simulink model "project"  (R2018b)
settings: Solver=VariableStepAuto  StartTime=0.0  StopTime=10.0  RelTol=1e-3
libraries: commutil2 x4
(part 1 of 2)
settings Model: Creator=Reza  LastModifiedBy=Rahmat

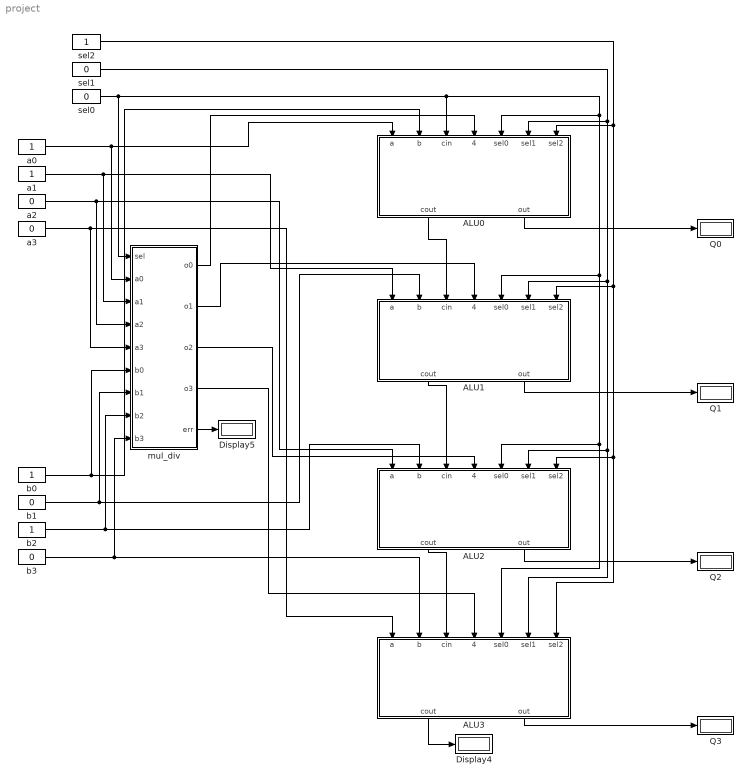
== system project ==
  ALU0 : Subsystem
  ALU1 : Subsystem
  ALU2 : Subsystem
  ALU3 : Subsystem
  Display4 : Display
  Display5 : Display
  Q{0..3} (4 alike) : Display
  a0 : Constant
  a1 : Constant
  a2 : Constant  Value=0
  a3 : Constant  Value=0
  b0 : Constant
  b1 : Constant  Value=0
  b2 : Constant
  b3 : Constant  Value=0
  mul_div : Subsystem
  sel0 : Constant  Value=0
  sel1 : Constant  Value=0
  sel2 : Constant
  wires:
  mul_div/1(o0) -> ALU0/4(mul_div)
  mul_div/2(o1) -> ALU1/4(mul_div)
  mul_div/3(o2) -> ALU2/4(mul_div)
  mul_div/4(o3) -> ALU3/4(mul_div)
  ALU0/1(cout) -> ALU1/3(cin)
  ALU1/1(cout) -> ALU2/3(cin)
  ALU2/1(cout) -> ALU3/3(cin)
  ALU0/2(out) -> Q0/1
  ALU1/2(out) -> Q1/1
  ALU2/2(out) -> Q2/1
  ALU3/2(out) -> Q3/1
  ALU3/1(cout) -> Display4/1
  mul_div/5(err) -> Display5/1
  sel0/1 -> mul_div/1(sel), ALU0/3(cin), ALU0/5(sel0), ALU1/5(sel0), ALU3/5(sel0), ALU2/5(sel0)
  sel1/1 -> ALU0/6(sel1), ALU1/6(sel1), ALU2/6(sel1), ALU3/6(sel1)
  sel2/1 -> ALU0/7(sel2), ALU1/7(sel2), ALU2/7(sel2), ALU3/7(sel2)
  a0/1 -> ALU0/1(a), mul_div/2(a0)
  a1/1 -> mul_div/3(a1), ALU1/1(a)
  a2/1 -> mul_div/4(a2), ALU2/1(a)
  a3/1 -> mul_div/5(a3), ALU3/1(a)
  b0/1 -> ALU0/2(b), mul_div/6(b0)
  b1/1 -> ALU1/2(b), mul_div/7(b1)
  b2/1 -> ALU2/2(b), mul_div/8(b2)
  b3/1 -> ALU3/2(b), mul_div/9(b3)

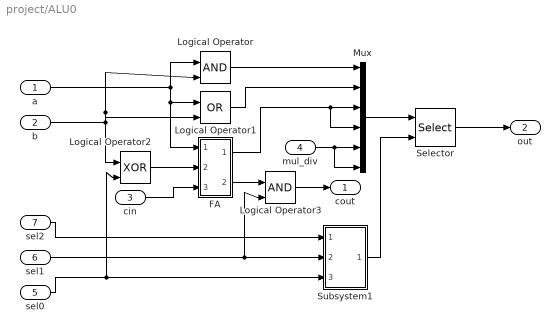
== system project/ALU0 ==
  a : Inport
  b : Inport  Port=2
  cin : Inport  Port=3
  mul_div : Inport  Port=4
  sel0 : Inport  Port=5
  sel1 : Inport  Port=6
  sel2 : Inport  Port=7
  FA : Subsystem
  Logical Operator : Logic  IconShape=distinctive  AllPortsSameDT=off  OutDataTypeStr=boolean
  Logical Operator1 : Logic  Operator=OR  IconShape=distinctive  AllPortsSameDT=off  OutDataTypeStr=boolean
  Logical Operator2 : Logic  Operator=XOR  IconShape=distinctive  AllPortsSameDT=off  OutDataTypeStr=boolean
  Logical Operator3 : Logic  IconShape=distinctive  AllPortsSameDT=off  OutDataTypeStr=boolean
  Mux : Mux  Inputs=6
  Selector : Selector  InputPortWidth=6  IndexOptions=Starting index (port)  Indices=[1 3]  OutputSizes=1
  Subsystem1 : Subsystem
  cout : Outport
  out : Outport  Port=2
  wires:
  b/1 -> Logical Operator/2, Logical Operator1/2, Logical Operator2/1
  Mux/1 -> Selector/1
  sel1/1 -> Logical Operator3/2, Subsystem1/2(sel1)
  FA/1(Out2) -> Mux/3, Mux/4
  sel2/1 -> Subsystem1/1(sel2)
  Subsystem1/1(Out1) -> Selector/2
  a/1 -> FA/1(In2), Logical Operator1/1, Logical Operator/1
  cin/1 -> FA/3(In4)
  Logical Operator2/1 -> FA/2(In3)
  Selector/1 -> out/1
  sel0/1 -> Logical Operator2/2, Subsystem1/3(sel0)
  Logical Operator1/1 -> Mux/2
  Logical Operator/1 -> Mux/1
  mul_div/1 -> Mux/5, Mux/6
  FA/2(Out1) -> Logical Operator3/1
  Logical Operator3/1 -> cout/1

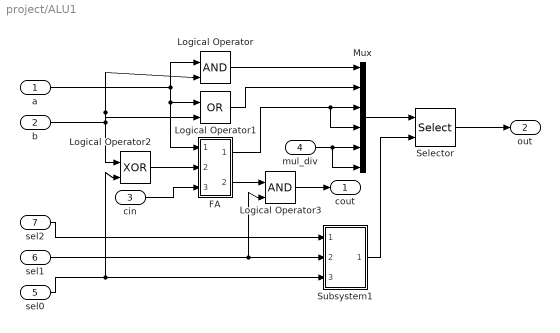
== system project/ALU1 ==
  a : Inport
  b : Inport  Port=2
  cin : Inport  Port=3
  mul_div : Inport  Port=4
  sel0 : Inport  Port=5
  sel1 : Inport  Port=6
  sel2 : Inport  Port=7
  FA : Subsystem
  Logical Operator : Logic  IconShape=distinctive  AllPortsSameDT=off  OutDataTypeStr=boolean
  Logical Operator1 : Logic  Operator=OR  IconShape=distinctive  AllPortsSameDT=off  OutDataTypeStr=boolean
  Logical Operator2 : Logic  Operator=XOR  IconShape=distinctive  AllPortsSameDT=off  OutDataTypeStr=boolean
  Logical Operator3 : Logic  IconShape=distinctive  AllPortsSameDT=off  OutDataTypeStr=boolean
  Mux : Mux  Inputs=6
  Selector : Selector  InputPortWidth=6  IndexOptions=Starting index (port)  Indices=[1 3]  OutputSizes=1
  Subsystem1 : Subsystem
  cout : Outport
  out : Outport  Port=2
  wires:
  b/1 -> Logical Operator/2, Logical Operator1/2, Logical Operator2/1
  Mux/1 -> Selector/1
  sel1/1 -> Logical Operator3/2, Subsystem1/2(sel1)
  FA/1(Out2) -> Mux/4, Mux/3
  sel2/1 -> Subsystem1/1(sel2)
  Subsystem1/1(Out1) -> Selector/2
  a/1 -> FA/1(In2), Logical Operator1/1, Logical Operator/1
  cin/1 -> FA/3(In4)
  sel0/1 -> Logical Operator2/2, Subsystem1/3(sel0)
  Logical Operator2/1 -> FA/2(In3)
  Selector/1 -> out/1
  Logical Operator/1 -> Mux/1
  Logical Operator1/1 -> Mux/2
  mul_div/1 -> Mux/6, Mux/5
  FA/2(Out1) -> Logical Operator3/1
  Logical Operator3/1 -> cout/1

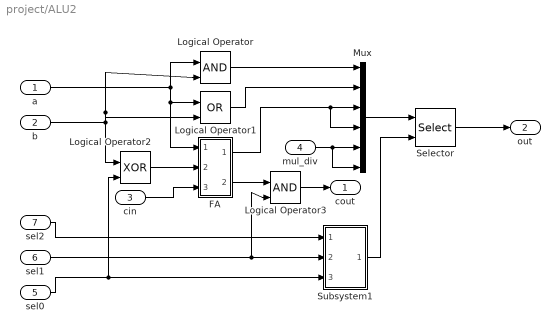
== system project/ALU2 ==
  a : Inport
  b : Inport  Port=2
  cin : Inport  Port=3
  mul_div : Inport  Port=4
  sel0 : Inport  Port=5
  sel1 : Inport  Port=6
  sel2 : Inport  Port=7
  FA : Subsystem
  Logical Operator : Logic  IconShape=distinctive  AllPortsSameDT=off  OutDataTypeStr=boolean
  Logical Operator1 : Logic  Operator=OR  IconShape=distinctive  AllPortsSameDT=off  OutDataTypeStr=boolean
  Logical Operator2 : Logic  Operator=XOR  IconShape=distinctive  AllPortsSameDT=off  OutDataTypeStr=boolean
  Logical Operator3 : Logic  IconShape=distinctive  AllPortsSameDT=off  OutDataTypeStr=boolean
  Mux : Mux  Inputs=6
  Selector : Selector  InputPortWidth=6  IndexOptions=Starting index (port)  Indices=[1 3]  OutputSizes=1
  Subsystem1 : Subsystem
  cout : Outport
  out : Outport  Port=2
  wires:
  b/1 -> Logical Operator/2, Logical Operator1/2, Logical Operator2/1
  Mux/1 -> Selector/1
  sel1/1 -> Logical Operator3/2, Subsystem1/2(sel1)
  FA/1(Out2) -> Mux/4, Mux/3
  sel2/1 -> Subsystem1/1(sel2)
  Subsystem1/1(Out1) -> Selector/2
  a/1 -> FA/1(In2), Logical Operator1/1, Logical Operator/1
  cin/1 -> FA/3(In4)
  sel0/1 -> Logical Operator2/2, Subsystem1/3(sel0)
  Logical Operator2/1 -> FA/2(In3)
  Selector/1 -> out/1
  Logical Operator1/1 -> Mux/2
  Logical Operator/1 -> Mux/1
  mul_div/1 -> Mux/5, Mux/6
  Logical Operator3/1 -> cout/1
  FA/2(Out1) -> Logical Operator3/1

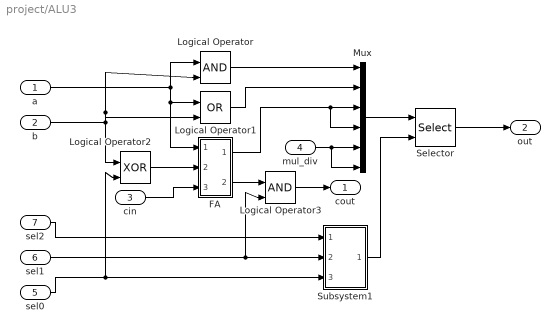
== system project/ALU3 ==
  a : Inport
  b : Inport  Port=2
  cin : Inport  Port=3
  mul_div : Inport  Port=4
  sel0 : Inport  Port=5
  sel1 : Inport  Port=6
  sel2 : Inport  Port=7
  FA : Subsystem
  Logical Operator : Logic  IconShape=distinctive  AllPortsSameDT=off  OutDataTypeStr=boolean
  Logical Operator1 : Logic  Operator=OR  IconShape=distinctive  AllPortsSameDT=off  OutDataTypeStr=boolean
  Logical Operator2 : Logic  Operator=XOR  IconShape=distinctive  AllPortsSameDT=off  OutDataTypeStr=boolean
  Logical Operator3 : Logic  IconShape=distinctive  AllPortsSameDT=off  OutDataTypeStr=boolean
  Mux : Mux  Inputs=6
  Selector : Selector  InputPortWidth=6  IndexOptions=Starting index (port)  Indices=[1 3]  OutputSizes=1
  Subsystem1 : Subsystem
  cout : Outport
  out : Outport  Port=2
  wires:
  b/1 -> Logical Operator/2, Logical Operator1/2, Logical Operator2/1
  Mux/1 -> Selector/1
  sel1/1 -> Logical Operator3/2, Subsystem1/2(sel1)
  FA/1(Out2) -> Mux/4, Mux/3
  sel2/1 -> Subsystem1/1(sel2)
  Subsystem1/1(Out1) -> Selector/2
  a/1 -> FA/1(In2), Logical Operator1/1, Logical Operator/1
  cin/1 -> FA/3(In4)
  sel0/1 -> Logical Operator2/2, Subsystem1/3(sel0)
  Logical Operator2/1 -> FA/2(In3)
  Selector/1 -> out/1
  Logical Operator1/1 -> Mux/2
  Logical Operator/1 -> Mux/1
  mul_div/1 -> Mux/6, Mux/5
  Logical Operator3/1 -> cout/1
  FA/2(Out1) -> Logical Operator3/1

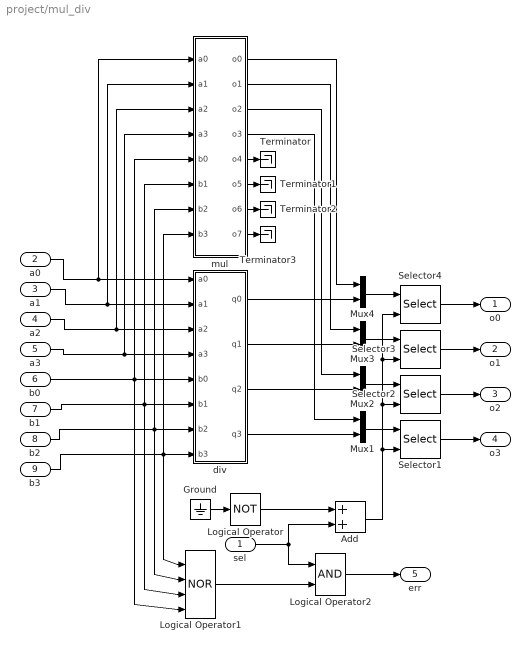
== system project/mul_div ==
  sel : Inport
  a0 : Inport  Port=2
  a1 : Inport  Port=3
  a2 : Inport  Port=4
  a3 : Inport  Port=5
  b0 : Inport  Port=6
  b1 : Inport  Port=7
  b2 : Inport  Port=8
  b3 : Inport  Port=9
  Add : Sum
  Ground : Ground
  Logical Operator : Logic  Operator=NOT  IconShape=distinctive  AllPortsSameDT=off  OutDataTypeStr=boolean
  Logical Operator1 : Logic  Operator=NOR  Inputs=4  IconShape=distinctive  AllPortsSameDT=off  OutDataTypeStr=boolean
  Logical Operator2 : Logic  IconShape=distinctive  AllPortsSameDT=off  OutDataTypeStr=boolean
  Mux{1..4} (4 alike) : Mux  Inputs=2
  Selector{1..4} (4 alike) : Selector  InputPortWidth=2  IndexOptions=Starting index (port)  Indices=[1 3]  OutputSizes=1
  Terminator{,1..3} (4 alike) : Terminator
  div : Subsystem
  mul : Subsystem
  o0 : Outport
  o1 : Outport  Port=2
  o2 : Outport  Port=3
  o3 : Outport  Port=4
  err : Outport  Port=5
  wires:
  Logical Operator/1 -> Add/1
  Ground/1 -> Logical Operator/1
  sel/1 -> Logical Operator2/1, Add/2
  Logical Operator2/1 -> err/1
  Mux1/1 -> Selector1/1
  Mux2/1 -> Selector2/1
  Mux3/1 -> Selector3/1
  Mux4/1 -> Selector4/1
  div/4(q3) -> Mux1/2
  div/3(q2) -> Mux2/2
  div/1(q0) -> Mux4/2
  div/2(q1) -> Mux3/2
  mul/1(o0) -> Mux4/1
  mul/2(o1) -> Mux3/1
  mul/3(o2) -> Mux2/1
  mul/4(o3) -> Mux1/1
  mul/5(o4) -> Terminator/1
  mul/6(o5) -> Terminator1/1
  mul/7(o6) -> Terminator2/1
  mul/8(o7) -> Terminator3/1
  Add/1 -> Selector1/2, Selector2/2, Selector3/2, Selector4/2
  Selector4/1 -> o0/1
  Selector3/1 -> o1/1
  Selector2/1 -> o2/1
  Selector1/1 -> o3/1
  a1/1 -> mul/2(a1), div/2(a1)
  a2/1 -> mul/3(a2), div/3(a2)
  a3/1 -> mul/4(a3), div/4(a3)
  b0/1 -> mul/5(b0), Logical Operator1/4, div/5(b0)
  b2/1 -> Logical Operator1/2, mul/7(b2), div/7(b2)
  b3/1 -> mul/8(b3), Logical Operator1/1, div/8(b3)
  Logical Operator1/1 -> Logical Operator2/2
  a0/1 -> div/1(a0), mul/1(a0)
  b1/1 -> Logical Operator1/3, mul/6(b1), div/6(b1)

== system project/ALU0/FA ==
  In2 : Inport
  In3 : Inport  Port=2
  In4 : Inport  Port=3
  Logical Operator : Logic  Operator=XOR  IconShape=distinctive  AllPortsSameDT=off  OutDataTypeStr=boolean
  Logical Operator1 : Logic  Operator=XOR  IconShape=distinctive  AllPortsSameDT=off  OutDataTypeStr=boolean
  Logical Operator2 : Logic  IconShape=distinctive  AllPortsSameDT=off  OutDataTypeStr=boolean
  Logical Operator3 : Logic  IconShape=distinctive  AllPortsSameDT=off  OutDataTypeStr=boolean
  Logical Operator4 : Logic  Operator=OR  IconShape=distinctive  AllPortsSameDT=off  OutDataTypeStr=boolean
  Out2 : Outport
  Out1 : Outport  Port=2
  wires:
  In2/1 -> Logical Operator3/1, Logical Operator/1
  In3/1 -> Logical Operator3/2, Logical Operator/2
  Logical Operator/1 -> Logical Operator1/1, Logical Operator2/1
  Logical Operator1/1 -> Out2/1
  Logical Operator4/1 -> Out1/1
  Logical Operator2/1 -> Logical Operator4/1
  Logical Operator3/1 -> Logical Operator4/2
  In4/1 -> Logical Operator2/2, Logical Operator1/2

== system project/ALU0/Subsystem1 ==
  sel2 : Inport
  sel1 : Inport  Port=2
  sel0 : Inport  Port=3
  Add : Sum
  Bit to Integer Converter : commutil2/Bit to Integer Converter  nbits=3  bitOrder=MSB first  signedOutputValues=Unsigned  outDtype=Inherit via internal rule  outDtypeSigned=Inherit via internal rule
  Ground : Ground
  Logical Operator3 : Logic  Operator=NOT  IconShape=distinctive  AllPortsSameDT=off  OutDataTypeStr=boolean
  Mux1 : Mux  Inputs=3
  Out1 : Outport
  wires:
  sel0/1 -> Mux1/3
  Ground/1 -> Logical Operator3/1
  Bit to Integer Converter/1 -> Add/1
  sel1/1 -> Mux1/2
  Mux1/1 -> Bit to Integer Converter/1
  Add/1 -> Out1/1
  Logical Operator3/1 -> Add/2
  sel2/1 -> Mux1/1

== system project/ALU1/FA ==
  In2 : Inport
  In3 : Inport  Port=2
  In4 : Inport  Port=3
  Logical Operator : Logic  Operator=XOR  IconShape=distinctive  AllPortsSameDT=off  OutDataTypeStr=boolean
  Logical Operator1 : Logic  Operator=XOR  IconShape=distinctive  AllPortsSameDT=off  OutDataTypeStr=boolean
  Logical Operator2 : Logic  IconShape=distinctive  AllPortsSameDT=off  OutDataTypeStr=boolean
  Logical Operator3 : Logic  IconShape=distinctive  AllPortsSameDT=off  OutDataTypeStr=boolean
  Logical Operator4 : Logic  Operator=OR  IconShape=distinctive  AllPortsSameDT=off  OutDataTypeStr=boolean
  Out2 : Outport
  Out1 : Outport  Port=2
  wires:
  Logical Operator2/1 -> Logical Operator4/1
  Logical Operator3/1 -> Logical Operator4/2
  Logical Operator1/1 -> Out2/1
  In4/1 -> Logical Operator2/2, Logical Operator1/2
  In3/1 -> Logical Operator3/2, Logical Operator/2
  In2/1 -> Logical Operator3/1, Logical Operator/1
  Logical Operator/1 -> Logical Operator1/1, Logical Operator2/1
  Logical Operator4/1 -> Out1/1

== system project/ALU1/Subsystem1 ==
  sel2 : Inport
  sel1 : Inport  Port=2
  sel0 : Inport  Port=3
  Add : Sum
  Bit to Integer Converter : commutil2/Bit to Integer Converter  nbits=3  bitOrder=MSB first  signedOutputValues=Unsigned  outDtype=Inherit via internal rule  outDtypeSigned=Inherit via internal rule
  Ground : Ground
  Logical Operator3 : Logic  Operator=NOT  IconShape=distinctive  AllPortsSameDT=off  OutDataTypeStr=boolean
  Mux1 : Mux  Inputs=3
  Out1 : Outport
  wires:
  sel0/1 -> Mux1/3
  Ground/1 -> Logical Operator3/1
  Bit to Integer Converter/1 -> Add/1
  sel1/1 -> Mux1/2
  Mux1/1 -> Bit to Integer Converter/1
  Add/1 -> Out1/1
  Logical Operator3/1 -> Add/2
  sel2/1 -> Mux1/1

== system project/ALU2/FA ==
  In2 : Inport
  In3 : Inport  Port=2
  In4 : Inport  Port=3
  Logical Operator : Logic  Operator=XOR  IconShape=distinctive  AllPortsSameDT=off  OutDataTypeStr=boolean
  Logical Operator1 : Logic  Operator=XOR  IconShape=distinctive  AllPortsSameDT=off  OutDataTypeStr=boolean
  Logical Operator2 : Logic  IconShape=distinctive  AllPortsSameDT=off  OutDataTypeStr=boolean
  Logical Operator3 : Logic  IconShape=distinctive  AllPortsSameDT=off  OutDataTypeStr=boolean
  Logical Operator4 : Logic  Operator=OR  IconShape=distinctive  AllPortsSameDT=off  OutDataTypeStr=boolean
  Out2 : Outport
  Out1 : Outport  Port=2
  wires:
  Logical Operator2/1 -> Logical Operator4/1
  Logical Operator3/1 -> Logical Operator4/2
  Logical Operator1/1 -> Out2/1
  In4/1 -> Logical Operator2/2, Logical Operator1/2
  In3/1 -> Logical Operator3/2, Logical Operator/2
  In2/1 -> Logical Operator3/1, Logical Operator/1
  Logical Operator/1 -> Logical Operator1/1, Logical Operator2/1
  Logical Operator4/1 -> Out1/1

== system project/ALU2/Subsystem1 ==
  sel2 : Inport
  sel1 : Inport  Port=2
  sel0 : Inport  Port=3
  Add : Sum
  Bit to Integer Converter : commutil2/Bit to Integer Converter  nbits=3  bitOrder=MSB first  signedOutputValues=Unsigned  outDtype=Inherit via internal rule  outDtypeSigned=Inherit via internal rule
  Ground : Ground
  Logical Operator3 : Logic  Operator=NOT  IconShape=distinctive  AllPortsSameDT=off  OutDataTypeStr=boolean
  Mux1 : Mux  Inputs=3
  Out1 : Outport
  wires:
  sel0/1 -> Mux1/3
  Ground/1 -> Logical Operator3/1
  Bit to Integer Converter/1 -> Add/1
  sel1/1 -> Mux1/2
  Mux1/1 -> Bit to Integer Converter/1
  Add/1 -> Out1/1
  Logical Operator3/1 -> Add/2
  sel2/1 -> Mux1/1

== system project/ALU3/FA ==
  In2 : Inport
  In3 : Inport  Port=2
  In4 : Inport  Port=3
  Logical Operator : Logic  Operator=XOR  IconShape=distinctive  AllPortsSameDT=off  OutDataTypeStr=boolean
  Logical Operator1 : Logic  Operator=XOR  IconShape=distinctive  AllPortsSameDT=off  OutDataTypeStr=boolean
  Logical Operator2 : Logic  IconShape=distinctive  AllPortsSameDT=off  OutDataTypeStr=boolean
  Logical Operator3 : Logic  IconShape=distinctive  AllPortsSameDT=off  OutDataTypeStr=boolean
  Logical Operator4 : Logic  Operator=OR  IconShape=distinctive  AllPortsSameDT=off  OutDataTypeStr=boolean
  Out2 : Outport
  Out1 : Outport  Port=2
  wires:
  Logical Operator2/1 -> Logical Operator4/1
  Logical Operator3/1 -> Logical Operator4/2
  Logical Operator1/1 -> Out2/1
  In4/1 -> Logical Operator2/2, Logical Operator1/2
  In3/1 -> Logical Operator3/2, Logical Operator/2
  In2/1 -> Logical Operator3/1, Logical Operator/1
  Logical Operator/1 -> Logical Operator1/1, Logical Operator2/1
  Logical Operator4/1 -> Out1/1

== system project/ALU3/Subsystem1 ==
  sel2 : Inport
  sel1 : Inport  Port=2
  sel0 : Inport  Port=3
  Add : Sum
  Bit to Integer Converter : commutil2/Bit to Integer Converter  nbits=3  bitOrder=MSB first  signedOutputValues=Unsigned  outDtype=Inherit via internal rule  outDtypeSigned=Inherit via internal rule
  Ground : Ground
  Logical Operator3 : Logic  Operator=NOT  IconShape=distinctive  AllPortsSameDT=off  OutDataTypeStr=boolean
  Mux1 : Mux  Inputs=3
  Out1 : Outport
  wires:
  sel0/1 -> Mux1/3
  Ground/1 -> Logical Operator3/1
  Bit to Integer Converter/1 -> Add/1
  sel1/1 -> Mux1/2
  Mux1/1 -> Bit to Integer Converter/1
  Add/1 -> Out1/1
  Logical Operator3/1 -> Add/2
  sel2/1 -> Mux1/1

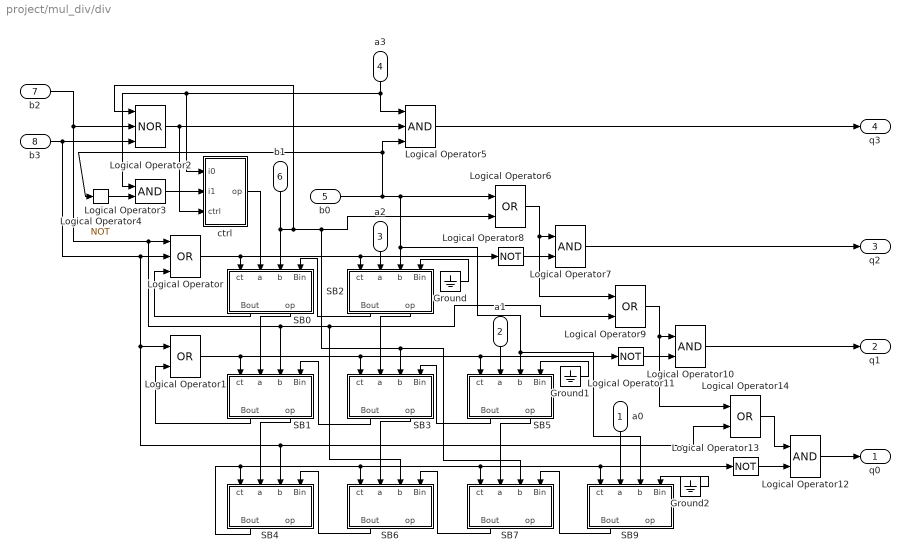
== system project/mul_div/div ==
  a0 : Inport
  a1 : Inport  Port=2
  a2 : Inport  Port=3
  a3 : Inport  Port=4
  b0 : Inport  Port=5
  b1 : Inport  Port=6
  b2 : Inport  Port=7
  b3 : Inport  Port=8
  Ground : Ground
  Ground1 : Ground
  Ground2 : Ground
  Logical Operator : Logic  Operator=OR  Inputs=3  IconShape=distinctive  AllPortsSameDT=off  OutDataTypeStr=boolean
  Logical Operator{1,6,9,14} (4 alike) : Logic  Operator=OR  IconShape=distinctive  AllPortsSameDT=off  OutDataTypeStr=boolean
  Logical Operator{3,7,10,12} (4 alike) : Logic  IconShape=distinctive  AllPortsSameDT=off  OutDataTypeStr=boolean
  Logical Operator{4,8,11,13} (4 alike) : Logic  Operator=NOT  IconShape=distinctive  AllPortsSameDT=off  OutDataTypeStr=boolean
  Logical Operator2 : Logic  Operator=NOR  Inputs=3  IconShape=distinctive  AllPortsSameDT=off  OutDataTypeStr=boolean
  Logical Operator5 : Logic  Inputs=3  IconShape=distinctive  AllPortsSameDT=off  OutDataTypeStr=boolean
  SB0 : Subsystem
  SB1 : Subsystem
  SB2 : Subsystem
  SB3 : Subsystem
  SB4 : Subsystem
  SB5 : Subsystem
  SB6 : Subsystem
  SB7 : Subsystem
  SB9 : Subsystem
  ctrl : Subsystem
  q0 : Outport
  q1 : Outport  Port=2
  q2 : Outport  Port=3
  q3 : Outport  Port=4
  wires:
  a2/1 -> SB2/2(a)
  a3/1 -> Logical Operator5/1, ctrl/1(i0), Logical Operator3/1
  b0/1 -> Logical Operator4/1, Logical Operator5/3, SB9/3(b), SB5/3(b), SB2/3(b), Logical Operator6/1
  Ground1/1 -> SB5/4(Bin)
  ctrl/1(op) -> SB0/2(a)
  Logical Operator9/1 -> Logical Operator14/1, Logical Operator10/1
  Logical Operator8/1 -> Logical Operator7/2
  Logical Operator11/1 -> Logical Operator10/2
  b3/1 -> SB4/3(b), Logical Operator14/2, Logical Operator1/1, Logical Operator/2, Logical Operator2/3
  SB6/1(Bout) -> SB4/4(Bin)
  b1/1 -> SB0/3(b), Logical Operator2/1, SB7/3(b), SB3/3(b), Logical Operator6/2
  b2/1 -> SB6/3(b), Logical Operator9/2, SB1/3(b), Logical Operator/1, Logical Operator2/2
  SB0/1(Bout) -> Logical Operator/3
  SB4/1(Bout) -> Logical Operator13/1, SB9/1(ct), SB7/1(ct), SB6/1(ct), SB4/1(ct)
  Logical Operator10/1 -> q1/1
  Logical Operator3/1 -> ctrl/2(i1)
  Logical Operator2/1 -> Logical Operator5/2, ctrl/3(ctrl)
  Logical Operator7/1 -> q2/1
  Logical Operator6/1 -> Logical Operator7/1, Logical Operator9/1
  SB5/2(op) -> SB7/2(a)
  Ground/1 -> SB2/4(Bin)
  Logical Operator5/1 -> q3/1
  SB2/2(op) -> SB3/2(a)
  Logical Operator/1 -> Logical Operator8/1, SB2/1(ct), SB0/1(ct)
  Logical Operator12/1 -> q0/1
  Logical Operator1/1 -> SB3/1(ct), Logical Operator11/1, SB5/1(ct), SB1/1(ct)
  SB3/2(op) -> SB6/2(a)
  SB1/2(op) -> SB4/2(a)
  a1/1 -> SB5/2(a)
  SB3/1(Bout) -> SB1/4(Bin)
  SB5/1(Bout) -> SB3/4(Bin)
  SB2/1(Bout) -> SB0/4(Bin)
  SB9/1(Bout) -> SB7/4(Bin)
  SB1/1(Bout) -> Logical Operator1/2
  Logical Operator4/1 -> Logical Operator3/2
  a0/1 -> SB9/2(a)
  Logical Operator13/1 -> Logical Operator12/2
  Logical Operator14/1 -> Logical Operator12/1
  SB7/1(Bout) -> SB6/4(Bin)
  SB0/2(op) -> SB1/2(a)
  Ground2/1 -> SB9/4(Bin)

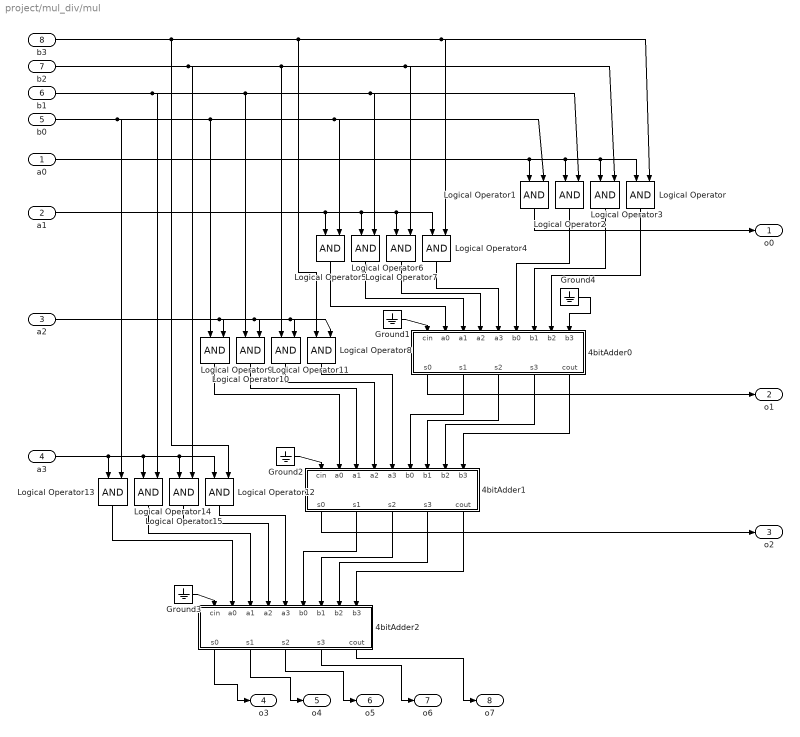
== system project/mul_div/mul ==
  a0 : Inport
  a1 : Inport  Port=2
  a2 : Inport  Port=3
  a3 : Inport  Port=4
  b0 : Inport  Port=5
  b1 : Inport  Port=6
  b2 : Inport  Port=7
  b3 : Inport  Port=8
  4bitAdder0 : Subsystem
  4bitAdder1 : Subsystem
  4bitAdder2 : Subsystem
  Ground{1..4} (4 alike) : Ground
  Logical Operator{,1..15} (16 alike) : Logic  IconShape=distinctive  AllPortsSameDT=off  OutDataTypeStr=boolean
  o0 : Outport
  o1 : Outport  Port=2
  o2 : Outport  Port=3
  o3 : Outport  Port=4
  o4 : Outport  Port=5
  o5 : Outport  Port=6
  o6 : Outport  Port=7
  o7 : Outport  Port=8
  wires:
  4bitAdder0/3(s2) -> 4bitAdder1/7(b1)
  b0/1 -> Logical Operator1/2, Logical Operator5/2, Logical Operator9/1, Logical Operator13/2
  Ground3/1 -> 4bitAdder2/1(cin)
  b1/1 -> Logical Operator2/2, Logical Operator6/2, Logical Operator10/1, Logical Operator14/2
  4bitAdder2/1(s0) -> o3/1
  Logical Operator12/1 -> 4bitAdder2/5(a3)
  Logical Operator9/1 -> 4bitAdder1/2(a0)
  a1/1 -> Logical Operator5/1, Logical Operator6/1, Logical Operator7/1, Logical Operator4/1
  Ground1/1 -> 4bitAdder0/1(cin)
  4bitAdder0/5(cout) -> 4bitAdder1/9(b3)
  Logical Operator14/1 -> 4bitAdder2/3(a1)
  Logical Operator5/1 -> 4bitAdder0/2(a0)
  4bitAdder2/5(cout) -> o7/1
  b2/1 -> Logical Operator3/2, Logical Operator7/2, Logical Operator11/1, Logical Operator15/2
  4bitAdder2/4(s3) -> o6/1
  Logical Operator8/1 -> 4bitAdder1/5(a3)
  Ground2/1 -> 4bitAdder1/1(cin)
  b3/1 -> Logical Operator/2, Logical Operator4/2, Logical Operator8/1, Logical Operator12/2
  4bitAdder2/2(s1) -> o4/1
  4bitAdder0/4(s3) -> 4bitAdder1/8(b2)
  4bitAdder1/4(s3) -> 4bitAdder2/8(b2)
  a3/1 -> Logical Operator13/1, Logical Operator14/1, Logical Operator15/1, Logical Operator12/1
  Logical Operator1/1 -> o0/1
  4bitAdder0/2(s1) -> 4bitAdder1/6(b0)
  4bitAdder1/2(s1) -> 4bitAdder2/6(b0)
  a2/1 -> Logical Operator9/2, Logical Operator10/2, Logical Operator11/2, Logical Operator8/2
  a0/1 -> Logical Operator1/1, Logical Operator2/1, Logical Operator3/1, Logical Operator/1
  4bitAdder1/3(s2) -> 4bitAdder2/7(b1)
  4bitAdder1/5(cout) -> 4bitAdder2/9(b3)
  Logical Operator15/1 -> 4bitAdder2/4(a2)
  4bitAdder0/1(s0) -> o1/1
  4bitAdder1/1(s0) -> o2/1
  Logical Operator13/1 -> 4bitAdder2/2(a0)
  Logical Operator7/1 -> 4bitAdder0/4(a2)
  Logical Operator11/1 -> 4bitAdder1/4(a2)
  Logical Operator10/1 -> 4bitAdder1/3(a1)
  4bitAdder2/3(s2) -> o5/1
  Logical Operator4/1 -> 4bitAdder0/5(a3)
  Logical Operator6/1 -> 4bitAdder0/3(a1)
  Logical Operator2/1 -> 4bitAdder0/6(b0)
  Logical Operator3/1 -> 4bitAdder0/7(b1)
  Logical Operator/1 -> 4bitAdder0/8(b2)
  Ground4/1 -> 4bitAdder0/9(b3)

== system project/mul_div/div/SB0 ==
  ct : Inport
  a : Inport  Port=2
  b : Inport  Port=3
  Bin : Inport  Port=4
  FS : Subsystem
  ctrl : Subsystem
  Bout : Outport
  op : Outport  Port=2
  wires:
  a/1 -> ctrl/2(i1), FS/1(a)
  ctrl/1(op) -> op/1
  ct/1 -> ctrl/3(ctrl)
  Bin/1 -> FS/3(Bin)
  FS/2(D) -> ctrl/1(i0)
  b/1 -> FS/2(b)
  FS/1(Bout) -> Bout/1

== system project/mul_div/div/SB1 ==
  ct : Inport
  a : Inport  Port=2
  b : Inport  Port=3
  Bin : Inport  Port=4
  FS : Subsystem
  ctrl : Subsystem
  Bout : Outport
  op : Outport  Port=2
  wires:
  a/1 -> ctrl/2(i1), FS/1(a)
  ctrl/1(op) -> op/1
  ct/1 -> ctrl/3(ctrl)
  Bin/1 -> FS/3(Bin)
  FS/2(D) -> ctrl/1(i0)
  b/1 -> FS/2(b)
  FS/1(Bout) -> Bout/1

== system project/mul_div/div/SB2 ==
  ct : Inport
  a : Inport  Port=2
  b : Inport  Port=3
  Bin : Inport  Port=4
  FS : Subsystem
  ctrl : Subsystem
  Bout : Outport
  op : Outport  Port=2
  wires:
  a/1 -> ctrl/2(i1), FS/1(a)
  ctrl/1(op) -> op/1
  ct/1 -> ctrl/3(ctrl)
  Bin/1 -> FS/3(Bin)
  FS/2(D) -> ctrl/1(i0)
  b/1 -> FS/2(b)
  FS/1(Bout) -> Bout/1

== system project/mul_div/div/SB3 ==
  ct : Inport
  a : Inport  Port=2
  b : Inport  Port=3
  Bin : Inport  Port=4
  FS : Subsystem
  ctrl : Subsystem
  Bout : Outport
  op : Outport  Port=2
  wires:
  a/1 -> ctrl/2(i1), FS/1(a)
  ctrl/1(op) -> op/1
  ct/1 -> ctrl/3(ctrl)
  Bin/1 -> FS/3(Bin)
  FS/2(D) -> ctrl/1(i0)
  b/1 -> FS/2(b)
  FS/1(Bout) -> Bout/1

== system project/mul_div/div/SB4 ==
  ct : Inport
  a : Inport  Port=2
  b : Inport  Port=3
  Bin : Inport  Port=4
  FS : Subsystem
  ctrl : Subsystem
  Bout : Outport
  op : Outport  Port=2
  wires:
  a/1 -> ctrl/2(i1), FS/1(a)
  ctrl/1(op) -> op/1
  ct/1 -> ctrl/3(ctrl)
  Bin/1 -> FS/3(Bin)
  FS/2(D) -> ctrl/1(i0)
  b/1 -> FS/2(b)
  FS/1(Bout) -> Bout/1

== system project/mul_div/div/SB5 ==
  ct : Inport
  a : Inport  Port=2
  b : Inport  Port=3
  Bin : Inport  Port=4
  FS : Subsystem
  ctrl : Subsystem
  Bout : Outport
  op : Outport  Port=2
  wires:
  a/1 -> ctrl/2(i1), FS/1(a)
  ctrl/1(op) -> op/1
  ct/1 -> ctrl/3(ctrl)
  Bin/1 -> FS/3(Bin)
  FS/2(D) -> ctrl/1(i0)
  b/1 -> FS/2(b)
  FS/1(Bout) -> Bout/1

== system project/mul_div/div/SB6 ==
  ct : Inport
  a : Inport  Port=2
  b : Inport  Port=3
  Bin : Inport  Port=4
  FS : Subsystem
  ctrl : Subsystem
  Bout : Outport
  op : Outport  Port=2
  wires:
  a/1 -> ctrl/2(i1), FS/1(a)
  ctrl/1(op) -> op/1
  ct/1 -> ctrl/3(ctrl)
  Bin/1 -> FS/3(Bin)
  FS/2(D) -> ctrl/1(i0)
  b/1 -> FS/2(b)
  FS/1(Bout) -> Bout/1

== system project/mul_div/div/SB7 ==
  ct : Inport
  a : Inport  Port=2
  b : Inport  Port=3
  Bin : Inport  Port=4
  FS : Subsystem
  ctrl : Subsystem
  Bout : Outport
  op : Outport  Port=2
  wires:
  a/1 -> ctrl/2(i1), FS/1(a)
  ctrl/1(op) -> op/1
  ct/1 -> ctrl/3(ctrl)
  Bin/1 -> FS/3(Bin)
  FS/2(D) -> ctrl/1(i0)
  b/1 -> FS/2(b)
  FS/1(Bout) -> Bout/1

== system project/mul_div/div/SB9 ==
  ct : Inport
  a : Inport  Port=2
  b : Inport  Port=3
  Bin : Inport  Port=4
  FS : Subsystem
  ctrl : Subsystem
  Bout : Outport
  op : Outport  Port=2
  wires:
  a/1 -> ctrl/2(i1), FS/1(a)
  ctrl/1(op) -> op/1
  ct/1 -> ctrl/3(ctrl)
  Bin/1 -> FS/3(Bin)
  FS/2(D) -> ctrl/1(i0)
  b/1 -> FS/2(b)
  FS/1(Bout) -> Bout/1

== system project/mul_div/div/ctrl ==
  i0 : Inport
  i1 : Inport  Port=2
  ctrl : Inport  Port=3
  Logical Operator : Logic  IconShape=distinctive  AllPortsSameDT=off  OutDataTypeStr=boolean
  Logical Operator1 : Logic  IconShape=distinctive  AllPortsSameDT=off  OutDataTypeStr=boolean
  Logical Operator2 : Logic  Operator=OR  IconShape=distinctive  AllPortsSameDT=off  OutDataTypeStr=boolean
  Logical Operator3 : Logic  Operator=NOT  IconShape=distinctive  AllPortsSameDT=off  OutDataTypeStr=boolean
  op : Outport
  wires:
  ctrl/1 -> Logical Operator3/1, Logical Operator1/2
  Logical Operator2/1 -> op/1
  Logical Operator3/1 -> Logical Operator/2
  i1/1 -> Logical Operator1/1
  i0/1 -> Logical Operator/1
  Logical Operator/1 -> Logical Operator2/1
  Logical Operator1/1 -> Logical Operator2/2

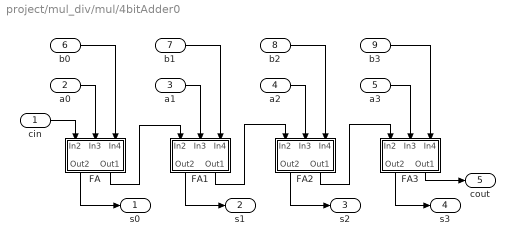
== system project/mul_div/mul/4bitAdder0 ==
  cin : Inport
  a0 : Inport  Port=2
  a1 : Inport  Port=3
  a2 : Inport  Port=4
  a3 : Inport  Port=5
  b0 : Inport  Port=6
  b1 : Inport  Port=7
  b2 : Inport  Port=8
  b3 : Inport  Port=9
  FA : Subsystem
  FA1 : Subsystem
  FA2 : Subsystem
  FA3 : Subsystem
  s0 : Outport
  s1 : Outport  Port=2
  s2 : Outport  Port=3
  s3 : Outport  Port=4
  cout : Outport  Port=5
  wires:
  a2/1 -> FA2/2(In3)
  a0/1 -> FA/2(In3)
  FA2/2(Out1) -> FA3/1(In2)
  b2/1 -> FA2/3(In4)
  b3/1 -> FA3/3(In4)
  cin/1 -> FA/1(In2)
  a3/1 -> FA3/2(In3)
  FA2/1(Out2) -> s2/1
  FA3/1(Out2) -> s3/1
  FA/1(Out2) -> s0/1
  b0/1 -> FA/3(In4)
  a1/1 -> FA1/2(In3)
  FA1/1(Out2) -> s1/1
  FA/2(Out1) -> FA1/1(In2)
  b1/1 -> FA1/3(In4)
  FA1/2(Out1) -> FA2/1(In2)
  FA3/2(Out1) -> cout/1

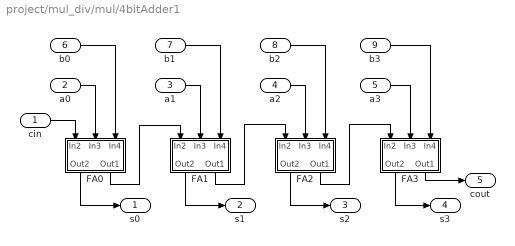
== system project/mul_div/mul/4bitAdder1 ==
  cin : Inport
  a0 : Inport  Port=2
  a1 : Inport  Port=3
  a2 : Inport  Port=4
  a3 : Inport  Port=5
  b0 : Inport  Port=6
  b1 : Inport  Port=7
  b2 : Inport  Port=8
  b3 : Inport  Port=9
  FA0 : Subsystem
  FA1 : Subsystem
  FA2 : Subsystem
  FA3 : Subsystem
  s0 : Outport
  s1 : Outport  Port=2
  s2 : Outport  Port=3
  s3 : Outport  Port=4
  cout : Outport  Port=5
  wires:
  a2/1 -> FA2/2(In3)
  a0/1 -> FA0/2(In3)
  FA2/2(Out1) -> FA3/1(In2)
  b2/1 -> FA2/3(In4)
  b3/1 -> FA3/3(In4)
  cin/1 -> FA0/1(In2)
  a3/1 -> FA3/2(In3)
  FA2/1(Out2) -> s2/1
  FA3/1(Out2) -> s3/1
  FA0/1(Out2) -> s0/1
  b0/1 -> FA0/3(In4)
  a1/1 -> FA1/2(In3)
  FA1/1(Out2) -> s1/1
  FA0/2(Out1) -> FA1/1(In2)
  b1/1 -> FA1/3(In4)
  FA1/2(Out1) -> FA2/1(In2)
  FA3/2(Out1) -> cout/1

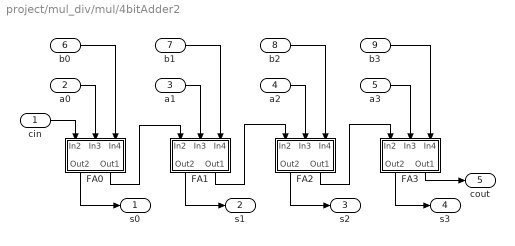
== system project/mul_div/mul/4bitAdder2 ==
  cin : Inport
  a0 : Inport  Port=2
  a1 : Inport  Port=3
  a2 : Inport  Port=4
  a3 : Inport  Port=5
  b0 : Inport  Port=6
  b1 : Inport  Port=7
  b2 : Inport  Port=8
  b3 : Inport  Port=9
  FA0 : Subsystem
  FA1 : Subsystem
  FA2 : Subsystem
  FA3 : Subsystem
  s0 : Outport
  s1 : Outport  Port=2
  s2 : Outport  Port=3
  s3 : Outport  Port=4
  cout : Outport  Port=5
  wires:
  a2/1 -> FA2/2(In3)
  a0/1 -> FA0/2(In3)
  FA2/2(Out1) -> FA3/1(In2)
  b2/1 -> FA2/3(In4)
  b3/1 -> FA3/3(In4)
  cin/1 -> FA0/1(In2)
  a3/1 -> FA3/2(In3)
  FA2/1(Out2) -> s2/1
  FA3/1(Out2) -> s3/1
  FA0/1(Out2) -> s0/1
  b0/1 -> FA0/3(In4)
  a1/1 -> FA1/2(In3)
  FA1/1(Out2) -> s1/1
  FA0/2(Out1) -> FA1/1(In2)
  b1/1 -> FA1/3(In4)
  FA1/2(Out1) -> FA2/1(In2)
  FA3/2(Out1) -> cout/1

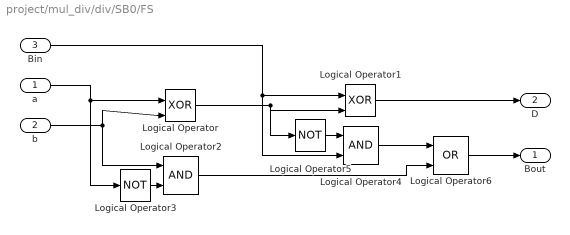
== system project/mul_div/div/SB0/FS ==
  a : Inport
  b : Inport  Port=2
  Bin : Inport  Port=3
  Logical Operator : Logic  Operator=XOR  IconShape=distinctive  AllPortsSameDT=off  OutDataTypeStr=boolean
  Logical Operator1 : Logic  Operator=XOR  IconShape=distinctive  AllPortsSameDT=off  OutDataTypeStr=boolean
  Logical Operator2 : Logic  IconShape=distinctive  AllPortsSameDT=off  OutDataTypeStr=boolean
  Logical Operator3 : Logic  Operator=NOT  IconShape=distinctive  AllPortsSameDT=off  OutDataTypeStr=boolean
  Logical Operator4 : Logic  IconShape=distinctive  AllPortsSameDT=off  OutDataTypeStr=boolean
  Logical Operator5 : Logic  Operator=NOT  IconShape=distinctive  AllPortsSameDT=off  OutDataTypeStr=boolean
  Logical Operator6 : Logic  Operator=OR  IconShape=distinctive  AllPortsSameDT=off  OutDataTypeStr=boolean
  Bout : Outport
  D : Outport  Port=2
  wires:
  Logical Operator2/1 -> Logical Operator6/2
  Bin/1 -> Logical Operator4/2, Logical Operator1/1
  Logical Operator3/1 -> Logical Operator2/2
  Logical Operator5/1 -> Logical Operator4/1
  b/1 -> Logical Operator/2, Logical Operator2/1
  Logical Operator6/1 -> Bout/1
  a/1 -> Logical Operator3/1, Logical Operator/1
  Logical Operator/1 -> Logical Operator5/1, Logical Operator1/2
  Logical Operator4/1 -> Logical Operator6/1
  Logical Operator1/1 -> D/1

== system project/mul_div/div/SB0/ctrl ==
  i0 : Inport
  i1 : Inport  Port=2
  ctrl : Inport  Port=3
  Logical Operator : Logic  IconShape=distinctive  AllPortsSameDT=off  OutDataTypeStr=boolean
  Logical Operator1 : Logic  IconShape=distinctive  AllPortsSameDT=off  OutDataTypeStr=boolean
  Logical Operator2 : Logic  Operator=OR  IconShape=distinctive  AllPortsSameDT=off  OutDataTypeStr=boolean
  Logical Operator3 : Logic  Operator=NOT  IconShape=distinctive  AllPortsSameDT=off  OutDataTypeStr=boolean
  op : Outport
  wires:
  ctrl/1 -> Logical Operator3/1, Logical Operator1/2
  Logical Operator2/1 -> op/1
  Logical Operator3/1 -> Logical Operator/2
  i1/1 -> Logical Operator1/1
  i0/1 -> Logical Operator/1
  Logical Operator/1 -> Logical Operator2/1
  Logical Operator1/1 -> Logical Operator2/2

== system project/mul_div/div/SB1/FS ==
  a : Inport
  b : Inport  Port=2
  Bin : Inport  Port=3
  Logical Operator : Logic  Operator=XOR  IconShape=distinctive  AllPortsSameDT=off  OutDataTypeStr=boolean
  Logical Operator1 : Logic  Operator=XOR  IconShape=distinctive  AllPortsSameDT=off  OutDataTypeStr=boolean
  Logical Operator2 : Logic  IconShape=distinctive  AllPortsSameDT=off  OutDataTypeStr=boolean
  Logical Operator3 : Logic  Operator=NOT  IconShape=distinctive  AllPortsSameDT=off  OutDataTypeStr=boolean
  Logical Operator4 : Logic  IconShape=distinctive  AllPortsSameDT=off  OutDataTypeStr=boolean
  Logical Operator5 : Logic  Operator=NOT  IconShape=distinctive  AllPortsSameDT=off  OutDataTypeStr=boolean
  Logical Operator6 : Logic  Operator=OR  IconShape=distinctive  AllPortsSameDT=off  OutDataTypeStr=boolean
  Bout : Outport
  D : Outport  Port=2
  wires:
  Logical Operator2/1 -> Logical Operator6/2
  Bin/1 -> Logical Operator4/2, Logical Operator1/1
  Logical Operator3/1 -> Logical Operator2/2
  Logical Operator5/1 -> Logical Operator4/1
  b/1 -> Logical Operator/2, Logical Operator2/1
  Logical Operator6/1 -> Bout/1
  a/1 -> Logical Operator3/1, Logical Operator/1
  Logical Operator/1 -> Logical Operator5/1, Logical Operator1/2
  Logical Operator4/1 -> Logical Operator6/1
  Logical Operator1/1 -> D/1

== system project/mul_div/div/SB1/ctrl ==
  i0 : Inport
  i1 : Inport  Port=2
  ctrl : Inport  Port=3
  Logical Operator : Logic  IconShape=distinctive  AllPortsSameDT=off  OutDataTypeStr=boolean
  Logical Operator1 : Logic  IconShape=distinctive  AllPortsSameDT=off  OutDataTypeStr=boolean
  Logical Operator2 : Logic  Operator=OR  IconShape=distinctive  AllPortsSameDT=off  OutDataTypeStr=boolean
  Logical Operator3 : Logic  Operator=NOT  IconShape=distinctive  AllPortsSameDT=off  OutDataTypeStr=boolean
  op : Outport
  wires:
  ctrl/1 -> Logical Operator3/1, Logical Operator1/2
  Logical Operator2/1 -> op/1
  Logical Operator3/1 -> Logical Operator/2
  i1/1 -> Logical Operator1/1
  i0/1 -> Logical Operator/1
  Logical Operator/1 -> Logical Operator2/1
  Logical Operator1/1 -> Logical Operator2/2

== system project/mul_div/div/SB2/FS ==
  a : Inport
  b : Inport  Port=2
  Bin : Inport  Port=3
  Logical Operator : Logic  Operator=XOR  IconShape=distinctive  AllPortsSameDT=off  OutDataTypeStr=boolean
  Logical Operator1 : Logic  Operator=XOR  IconShape=distinctive  AllPortsSameDT=off  OutDataTypeStr=boolean
  Logical Operator2 : Logic  IconShape=distinctive  AllPortsSameDT=off  OutDataTypeStr=boolean
  Logical Operator3 : Logic  Operator=NOT  IconShape=distinctive  AllPortsSameDT=off  OutDataTypeStr=boolean
  Logical Operator4 : Logic  IconShape=distinctive  AllPortsSameDT=off  OutDataTypeStr=boolean
  Logical Operator5 : Logic  Operator=NOT  IconShape=distinctive  AllPortsSameDT=off  OutDataTypeStr=boolean
  Logical Operator6 : Logic  Operator=OR  IconShape=distinctive  AllPortsSameDT=off  OutDataTypeStr=boolean
  Bout : Outport
  D : Outport  Port=2
  wires:
  Logical Operator2/1 -> Logical Operator6/2
  Bin/1 -> Logical Operator4/2, Logical Operator1/1
  Logical Operator3/1 -> Logical Operator2/2
  Logical Operator5/1 -> Logical Operator4/1
  b/1 -> Logical Operator/2, Logical Operator2/1
  Logical Operator6/1 -> Bout/1
  a/1 -> Logical Operator3/1, Logical Operator/1
  Logical Operator/1 -> Logical Operator5/1, Logical Operator1/2
  Logical Operator4/1 -> Logical Operator6/1
  Logical Operator1/1 -> D/1

== system project/mul_div/div/SB2/ctrl ==
  i0 : Inport
  i1 : Inport  Port=2
  ctrl : Inport  Port=3
  Logical Operator : Logic  IconShape=distinctive  AllPortsSameDT=off  OutDataTypeStr=boolean
  Logical Operator1 : Logic  IconShape=distinctive  AllPortsSameDT=off  OutDataTypeStr=boolean
  Logical Operator2 : Logic  Operator=OR  IconShape=distinctive  AllPortsSameDT=off  OutDataTypeStr=boolean
  Logical Operator3 : Logic  Operator=NOT  IconShape=distinctive  AllPortsSameDT=off  OutDataTypeStr=boolean
  op : Outport
  wires:
  ctrl/1 -> Logical Operator3/1, Logical Operator1/2
  Logical Operator2/1 -> op/1
  Logical Operator3/1 -> Logical Operator/2
  i1/1 -> Logical Operator1/1
  i0/1 -> Logical Operator/1
  Logical Operator/1 -> Logical Operator2/1
  Logical Operator1/1 -> Logical Operator2/2

== system project/mul_div/div/SB3/FS ==
  a : Inport
  b : Inport  Port=2
  Bin : Inport  Port=3
  Logical Operator : Logic  Operator=XOR  IconShape=distinctive  AllPortsSameDT=off  OutDataTypeStr=boolean
  Logical Operator1 : Logic  Operator=XOR  IconShape=distinctive  AllPortsSameDT=off  OutDataTypeStr=boolean
  Logical Operator2 : Logic  IconShape=distinctive  AllPortsSameDT=off  OutDataTypeStr=boolean
  Logical Operator3 : Logic  Operator=NOT  IconShape=distinctive  AllPortsSameDT=off  OutDataTypeStr=boolean
  Logical Operator4 : Logic  IconShape=distinctive  AllPortsSameDT=off  OutDataTypeStr=boolean
  Logical Operator5 : Logic  Operator=NOT  IconShape=distinctive  AllPortsSameDT=off  OutDataTypeStr=boolean
  Logical Operator6 : Logic  Operator=OR  IconShape=distinctive  AllPortsSameDT=off  OutDataTypeStr=boolean
  Bout : Outport
  D : Outport  Port=2
  wires:
  Logical Operator2/1 -> Logical Operator6/2
  Bin/1 -> Logical Operator4/2, Logical Operator1/1
  Logical Operator3/1 -> Logical Operator2/2
  Logical Operator5/1 -> Logical Operator4/1
  b/1 -> Logical Operator/2, Logical Operator2/1
  Logical Operator6/1 -> Bout/1
  a/1 -> Logical Operator3/1, Logical Operator/1
  Logical Operator/1 -> Logical Operator5/1, Logical Operator1/2
  Logical Operator4/1 -> Logical Operator6/1
  Logical Operator1/1 -> D/1

== system project/mul_div/div/SB3/ctrl ==
  i0 : Inport
  i1 : Inport  Port=2
  ctrl : Inport  Port=3
  Logical Operator : Logic  IconShape=distinctive  AllPortsSameDT=off  OutDataTypeStr=boolean
  Logical Operator1 : Logic  IconShape=distinctive  AllPortsSameDT=off  OutDataTypeStr=boolean
  Logical Operator2 : Logic  Operator=OR  IconShape=distinctive  AllPortsSameDT=off  OutDataTypeStr=boolean
  Logical Operator3 : Logic  Operator=NOT  IconShape=distinctive  AllPortsSameDT=off  OutDataTypeStr=boolean
  op : Outport
  wires:
  ctrl/1 -> Logical Operator3/1, Logical Operator1/2
  Logical Operator2/1 -> op/1
  Logical Operator3/1 -> Logical Operator/2
  i1/1 -> Logical Operator1/1
  i0/1 -> Logical Operator/1
  Logical Operator/1 -> Logical Operator2/1
  Logical Operator1/1 -> Logical Operator2/2

== system project/mul_div/div/SB4/FS ==
  a : Inport
  b : Inport  Port=2
  Bin : Inport  Port=3
  Logical Operator : Logic  Operator=XOR  IconShape=distinctive  AllPortsSameDT=off  OutDataTypeStr=boolean
  Logical Operator1 : Logic  Operator=XOR  IconShape=distinctive  AllPortsSameDT=off  OutDataTypeStr=boolean
  Logical Operator2 : Logic  IconShape=distinctive  AllPortsSameDT=off  OutDataTypeStr=boolean
  Logical Operator3 : Logic  Operator=NOT  IconShape=distinctive  AllPortsSameDT=off  OutDataTypeStr=boolean
  Logical Operator4 : Logic  IconShape=distinctive  AllPortsSameDT=off  OutDataTypeStr=boolean
  Logical Operator5 : Logic  Operator=NOT  IconShape=distinctive  AllPortsSameDT=off  OutDataTypeStr=boolean
  Logical Operator6 : Logic  Operator=OR  IconShape=distinctive  AllPortsSameDT=off  OutDataTypeStr=boolean
  Bout : Outport
  D : Outport  Port=2
  wires:
  Logical Operator2/1 -> Logical Operator6/2
  Bin/1 -> Logical Operator4/2, Logical Operator1/1
  Logical Operator3/1 -> Logical Operator2/2
  Logical Operator5/1 -> Logical Operator4/1
  b/1 -> Logical Operator/2, Logical Operator2/1
  Logical Operator6/1 -> Bout/1
  a/1 -> Logical Operator3/1, Logical Operator/1
  Logical Operator/1 -> Logical Operator5/1, Logical Operator1/2
  Logical Operator4/1 -> Logical Operator6/1
  Logical Operator1/1 -> D/1

== system project/mul_div/div/SB4/ctrl ==
  i0 : Inport
  i1 : Inport  Port=2
  ctrl : Inport  Port=3
  Logical Operator : Logic  IconShape=distinctive  AllPortsSameDT=off  OutDataTypeStr=boolean
  Logical Operator1 : Logic  IconShape=distinctive  AllPortsSameDT=off  OutDataTypeStr=boolean
  Logical Operator2 : Logic  Operator=OR  IconShape=distinctive  AllPortsSameDT=off  OutDataTypeStr=boolean
  Logical Operator3 : Logic  Operator=NOT  IconShape=distinctive  AllPortsSameDT=off  OutDataTypeStr=boolean
  op : Outport
  wires:
  ctrl/1 -> Logical Operator3/1, Logical Operator1/2
  Logical Operator2/1 -> op/1
  Logical Operator3/1 -> Logical Operator/2
  i1/1 -> Logical Operator1/1
  i0/1 -> Logical Operator/1
  Logical Operator/1 -> Logical Operator2/1
  Logical Operator1/1 -> Logical Operator2/2

== system project/mul_div/div/SB5/FS ==
  a : Inport
  b : Inport  Port=2
  Bin : Inport  Port=3
  Logical Operator : Logic  Operator=XOR  IconShape=distinctive  AllPortsSameDT=off  OutDataTypeStr=boolean
  Logical Operator1 : Logic  Operator=XOR  IconShape=distinctive  AllPortsSameDT=off  OutDataTypeStr=boolean
  Logical Operator2 : Logic  IconShape=distinctive  AllPortsSameDT=off  OutDataTypeStr=boolean
  Logical Operator3 : Logic  Operator=NOT  IconShape=distinctive  AllPortsSameDT=off  OutDataTypeStr=boolean
  Logical Operator4 : Logic  IconShape=distinctive  AllPortsSameDT=off  OutDataTypeStr=boolean
  Logical Operator5 : Logic  Operator=NOT  IconShape=distinctive  AllPortsSameDT=off  OutDataTypeStr=boolean
  Logical Operator6 : Logic  Operator=OR  IconShape=distinctive  AllPortsSameDT=off  OutDataTypeStr=boolean
  Bout : Outport
  D : Outport  Port=2
  wires:
  Logical Operator2/1 -> Logical Operator6/2
  Bin/1 -> Logical Operator4/2, Logical Operator1/1
  Logical Operator3/1 -> Logical Operator2/2
  Logical Operator5/1 -> Logical Operator4/1
  b/1 -> Logical Operator/2, Logical Operator2/1
  Logical Operator6/1 -> Bout/1
  a/1 -> Logical Operator3/1, Logical Operator/1
  Logical Operator/1 -> Logical Operator5/1, Logical Operator1/2
  Logical Operator4/1 -> Logical Operator6/1
  Logical Operator1/1 -> D/1

== system project/mul_div/div/SB5/ctrl ==
  i0 : Inport
  i1 : Inport  Port=2
  ctrl : Inport  Port=3
  Logical Operator : Logic  IconShape=distinctive  AllPortsSameDT=off  OutDataTypeStr=boolean
  Logical Operator1 : Logic  IconShape=distinctive  AllPortsSameDT=off  OutDataTypeStr=boolean
  Logical Operator2 : Logic  Operator=OR  IconShape=distinctive  AllPortsSameDT=off  OutDataTypeStr=boolean
  Logical Operator3 : Logic  Operator=NOT  IconShape=distinctive  AllPortsSameDT=off  OutDataTypeStr=boolean
  op : Outport
  wires:
  ctrl/1 -> Logical Operator3/1, Logical Operator1/2
  Logical Operator2/1 -> op/1
  Logical Operator3/1 -> Logical Operator/2
  i1/1 -> Logical Operator1/1
  i0/1 -> Logical Operator/1
  Logical Operator/1 -> Logical Operator2/1
  Logical Operator1/1 -> Logical Operator2/2

== system project/mul_div/div/SB6/FS ==
  a : Inport
  b : Inport  Port=2
  Bin : Inport  Port=3
  Logical Operator : Logic  Operator=XOR  IconShape=distinctive  AllPortsSameDT=off  OutDataTypeStr=boolean
  Logical Operator1 : Logic  Operator=XOR  IconShape=distinctive  AllPortsSameDT=off  OutDataTypeStr=boolean
  Logical Operator2 : Logic  IconShape=distinctive  AllPortsSameDT=off  OutDataTypeStr=boolean
  Logical Operator3 : Logic  Operator=NOT  IconShape=distinctive  AllPortsSameDT=off  OutDataTypeStr=boolean
  Logical Operator4 : Logic  IconShape=distinctive  AllPortsSameDT=off  OutDataTypeStr=boolean
  Logical Operator5 : Logic  Operator=NOT  IconShape=distinctive  AllPortsSameDT=off  OutDataTypeStr=boolean
  Logical Operator6 : Logic  Operator=OR  IconShape=distinctive  AllPortsSameDT=off  OutDataTypeStr=boolean
  Bout : Outport
  D : Outport  Port=2
  wires:
  Logical Operator2/1 -> Logical Operator6/2
  Bin/1 -> Logical Operator4/2, Logical Operator1/1
  Logical Operator3/1 -> Logical Operator2/2
  Logical Operator5/1 -> Logical Operator4/1
  b/1 -> Logical Operator/2, Logical Operator2/1
  Logical Operator6/1 -> Bout/1
  a/1 -> Logical Operator3/1, Logical Operator/1
  Logical Operator/1 -> Logical Operator5/1, Logical Operator1/2
  Logical Operator4/1 -> Logical Operator6/1
  Logical Operator1/1 -> D/1

== system project/mul_div/div/SB6/ctrl ==
  i0 : Inport
  i1 : Inport  Port=2
  ctrl : Inport  Port=3
  Logical Operator : Logic  IconShape=distinctive  AllPortsSameDT=off  OutDataTypeStr=boolean
  Logical Operator1 : Logic  IconShape=distinctive  AllPortsSameDT=off  OutDataTypeStr=boolean
  Logical Operator2 : Logic  Operator=OR  IconShape=distinctive  AllPortsSameDT=off  OutDataTypeStr=boolean
  Logical Operator3 : Logic  Operator=NOT  IconShape=distinctive  AllPortsSameDT=off  OutDataTypeStr=boolean
  op : Outport
  wires:
  ctrl/1 -> Logical Operator3/1, Logical Operator1/2
  Logical Operator2/1 -> op/1
  Logical Operator3/1 -> Logical Operator/2
  i1/1 -> Logical Operator1/1
  i0/1 -> Logical Operator/1
  Logical Operator/1 -> Logical Operator2/1
  Logical Operator1/1 -> Logical Operator2/2

== system project/mul_div/div/SB7/FS ==
  a : Inport
  b : Inport  Port=2
  Bin : Inport  Port=3
  Logical Operator : Logic  Operator=XOR  IconShape=distinctive  AllPortsSameDT=off  OutDataTypeStr=boolean
  Logical Operator1 : Logic  Operator=XOR  IconShape=distinctive  AllPortsSameDT=off  OutDataTypeStr=boolean
  Logical Operator2 : Logic  IconShape=distinctive  AllPortsSameDT=off  OutDataTypeStr=boolean
  Logical Operator3 : Logic  Operator=NOT  IconShape=distinctive  AllPortsSameDT=off  OutDataTypeStr=boolean
  Logical Operator4 : Logic  IconShape=distinctive  AllPortsSameDT=off  OutDataTypeStr=boolean
  Logical Operator5 : Logic  Operator=NOT  IconShape=distinctive  AllPortsSameDT=off  OutDataTypeStr=boolean
  Logical Operator6 : Logic  Operator=OR  IconShape=distinctive  AllPortsSameDT=off  OutDataTypeStr=boolean
  Bout : Outport
  D : Outport  Port=2
  wires:
  Logical Operator2/1 -> Logical Operator6/2
  Bin/1 -> Logical Operator4/2, Logical Operator1/1
  Logical Operator3/1 -> Logical Operator2/2
  Logical Operator5/1 -> Logical Operator4/1
  b/1 -> Logical Operator/2, Logical Operator2/1
  Logical Operator6/1 -> Bout/1
  a/1 -> Logical Operator3/1, Logical Operator/1
  Logical Operator/1 -> Logical Operator5/1, Logical Operator1/2
  Logical Operator4/1 -> Logical Operator6/1
  Logical Operator1/1 -> D/1

== system project/mul_div/div/SB7/ctrl ==
  i0 : Inport
  i1 : Inport  Port=2
  ctrl : Inport  Port=3
  Logical Operator : Logic  IconShape=distinctive  AllPortsSameDT=off  OutDataTypeStr=boolean
  Logical Operator1 : Logic  IconShape=distinctive  AllPortsSameDT=off  OutDataTypeStr=boolean
  Logical Operator2 : Logic  Operator=OR  IconShape=distinctive  AllPortsSameDT=off  OutDataTypeStr=boolean
  Logical Operator3 : Logic  Operator=NOT  IconShape=distinctive  AllPortsSameDT=off  OutDataTypeStr=boolean
  op : Outport
  wires:
  ctrl/1 -> Logical Operator3/1, Logical Operator1/2
  Logical Operator2/1 -> op/1
  Logical Operator3/1 -> Logical Operator/2
  i1/1 -> Logical Operator1/1
  i0/1 -> Logical Operator/1
  Logical Operator/1 -> Logical Operator2/1
  Logical Operator1/1 -> Logical Operator2/2

== system project/mul_div/div/SB9/FS ==
  a : Inport
  b : Inport  Port=2
  Bin : Inport  Port=3
  Logical Operator : Logic  Operator=XOR  IconShape=distinctive  AllPortsSameDT=off  OutDataTypeStr=boolean
  Logical Operator1 : Logic  Operator=XOR  IconShape=distinctive  AllPortsSameDT=off  OutDataTypeStr=boolean
  Logical Operator2 : Logic  IconShape=distinctive  AllPortsSameDT=off  OutDataTypeStr=boolean
  Logical Operator3 : Logic  Operator=NOT  IconShape=distinctive  AllPortsSameDT=off  OutDataTypeStr=boolean
  Logical Operator4 : Logic  IconShape=distinctive  AllPortsSameDT=off  OutDataTypeStr=boolean
  Logical Operator5 : Logic  Operator=NOT  IconShape=distinctive  AllPortsSameDT=off  OutDataTypeStr=boolean
  Logical Operator6 : Logic  Operator=OR  IconShape=distinctive  AllPortsSameDT=off  OutDataTypeStr=boolean
  Bout : Outport
  D : Outport  Port=2
  wires:
  Logical Operator2/1 -> Logical Operator6/2
  Bin/1 -> Logical Operator4/2, Logical Operator1/1
  Logical Operator3/1 -> Logical Operator2/2
  Logical Operator5/1 -> Logical Operator4/1
  b/1 -> Logical Operator/2, Logical Operator2/1
  Logical Operator6/1 -> Bout/1
  a/1 -> Logical Operator3/1, Logical Operator/1
  Logical Operator/1 -> Logical Operator5/1, Logical Operator1/2
  Logical Operator4/1 -> Logical Operator6/1
  Logical Operator1/1 -> D/1

== system project/mul_div/div/SB9/ctrl ==
  i0 : Inport
  i1 : Inport  Port=2
  ctrl : Inport  Port=3
  Logical Operator : Logic  IconShape=distinctive  AllPortsSameDT=off  OutDataTypeStr=boolean
  Logical Operator1 : Logic  IconShape=distinctive  AllPortsSameDT=off  OutDataTypeStr=boolean
  Logical Operator2 : Logic  Operator=OR  IconShape=distinctive  AllPortsSameDT=off  OutDataTypeStr=boolean
  Logical Operator3 : Logic  Operator=NOT  IconShape=distinctive  AllPortsSameDT=off  OutDataTypeStr=boolean
  op : Outport
  wires:
  ctrl/1 -> Logical Operator3/1, Logical Operator1/2
  Logical Operator2/1 -> op/1
  Logical Operator3/1 -> Logical Operator/2
  i1/1 -> Logical Operator1/1
  i0/1 -> Logical Operator/1
  Logical Operator/1 -> Logical Operator2/1
  Logical Operator1/1 -> Logical Operator2/2

== system project/mul_div/mul/4bitAdder0/FA ==
  In2 : Inport
  In3 : Inport  Port=2
  In4 : Inport  Port=3
  Logical Operator : Logic  Operator=XOR  IconShape=distinctive  AllPortsSameDT=off  OutDataTypeStr=boolean
  Logical Operator1 : Logic  Operator=XOR  IconShape=distinctive  AllPortsSameDT=off  OutDataTypeStr=boolean
  Logical Operator2 : Logic  IconShape=distinctive  AllPortsSameDT=off  OutDataTypeStr=boolean
  Logical Operator3 : Logic  IconShape=distinctive  AllPortsSameDT=off  OutDataTypeStr=boolean
  Logical Operator4 : Logic  Operator=OR  IconShape=distinctive  AllPortsSameDT=off  OutDataTypeStr=boolean
  Out2 : Outport
  Out1 : Outport  Port=2
  wires:
  Logical Operator2/1 -> Logical Operator4/1
  Logical Operator3/1 -> Logical Operator4/2
  Logical Operator1/1 -> Out2/1
  In4/1 -> Logical Operator2/2, Logical Operator1/2
  In3/1 -> Logical Operator3/2, Logical Operator/2
  In2/1 -> Logical Operator3/1, Logical Operator/1
  Logical Operator/1 -> Logical Operator1/1, Logical Operator2/1
  Logical Operator4/1 -> Out1/1

== system project/mul_div/mul/4bitAdder0/FA1 ==
  In2 : Inport
  In3 : Inport  Port=2
  In4 : Inport  Port=3
  Logical Operator : Logic  Operator=XOR  IconShape=distinctive  AllPortsSameDT=off  OutDataTypeStr=boolean
  Logical Operator1 : Logic  Operator=XOR  IconShape=distinctive  AllPortsSameDT=off  OutDataTypeStr=boolean
  Logical Operator2 : Logic  IconShape=distinctive  AllPortsSameDT=off  OutDataTypeStr=boolean
  Logical Operator3 : Logic  IconShape=distinctive  AllPortsSameDT=off  OutDataTypeStr=boolean
  Logical Operator4 : Logic  Operator=OR  IconShape=distinctive  AllPortsSameDT=off  OutDataTypeStr=boolean
  Out2 : Outport
  Out1 : Outport  Port=2
  wires:
  Logical Operator2/1 -> Logical Operator4/1
  Logical Operator3/1 -> Logical Operator4/2
  Logical Operator1/1 -> Out2/1
  In4/1 -> Logical Operator2/2, Logical Operator1/2
  In3/1 -> Logical Operator3/2, Logical Operator/2
  In2/1 -> Logical Operator3/1, Logical Operator/1
  Logical Operator/1 -> Logical Operator1/1, Logical Operator2/1
  Logical Operator4/1 -> Out1/1
